simulink library "Driver_Open_Loop"  (R2026a)
settings: Solver=VariableStepAuto
undefined symbols (not defined in the file): Maneuver
libraries: simulink x3
Description:
  | Component of Simscape Vehicle Templates Library
  | 
  | Copyright 2018-2026 The MathWorks, Inc.
settings Model: Creator=smiller  LastModifiedBy=smiller

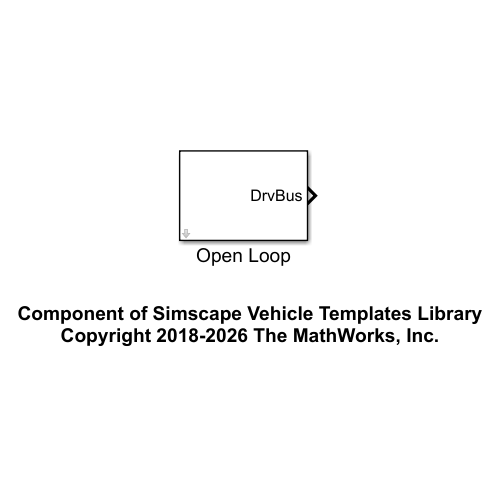
[thumbnail: Simulink's stored preview of the top-level diagram]
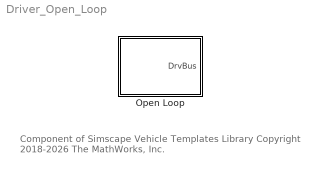
== system Driver_Open_Loop ==
  note: Component of Simscape Vehicle Templates Library
      | Copyright 2018-2026 The MathWorks, Inc.
  Open Loop : Subsystem  mask{Maneuver=Maneuver}
      mask init:
      | X = [0 0];
      | Y = [0 0];

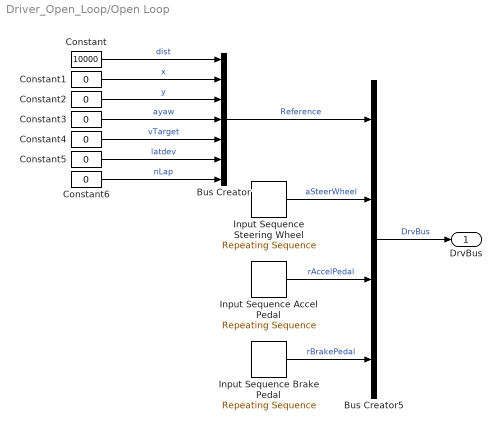
== system Driver_Open_Loop/Open Loop ==
  Bus Creator : BusCreator  Inputs=7
  Bus Creator5 : BusCreator  Inputs=4
  Constant : Constant  Value=10000
  Constant{1..6} (6 alike) : Constant  Value=0
  Input Sequence Accel Pedal : simulink/Sources/Repeating Sequence  rep_seq_t=Maneuver.Accel.t.Value  rep_seq_y=Maneuver.Accel.rPedal.Value
  Input Sequence Brake Pedal : simulink/Sources/Repeating Sequence  rep_seq_t=Maneuver.Brake.t.Value  rep_seq_y=Maneuver.Brake.rPedal.Value
  "Input Sequence Steering Wheel " : simulink/Sources/Repeating Sequence  rep_seq_t=Maneuver.Steer.t.Value  rep_seq_y=Maneuver.Steer.aWheel.Value
  DrvBus : Outport  VectorParamsAs1DForOutWhenUnconnected=off
  wires:
  Bus Creator5/1 -> DrvBus/1  "DrvBus"
  Input Sequence Brake Pedal/1 -> Bus Creator5/4  "rBrakePedal"
  "Input Sequence Steering Wheel "/1 -> Bus Creator5/2  "aSteerWheel"
  Input Sequence Accel Pedal/1 -> Bus Creator5/3  "rAccelPedal"
  Constant1/1 -> Bus Creator/2  "x"
  Constant5/1 -> Bus Creator/6  "latdev"
  Constant2/1 -> Bus Creator/3  "y"
  Constant3/1 -> Bus Creator/4  "ayaw"
  Constant4/1 -> Bus Creator/5  "vTarget"
  Bus Creator/1 -> Bus Creator5/1  "Reference"
  Constant/1 -> Bus Creator/1  "dist"
  Constant6/1 -> Bus Creator/7  "nLap"
